simulink model "constFeed"  (R2022a)
settings: Solver=VariableStepAuto  StartTime=0.0  StopTime=240  RelTol=1e-3
settings Model: Creator=tomok  LastModifiedBy=tomok

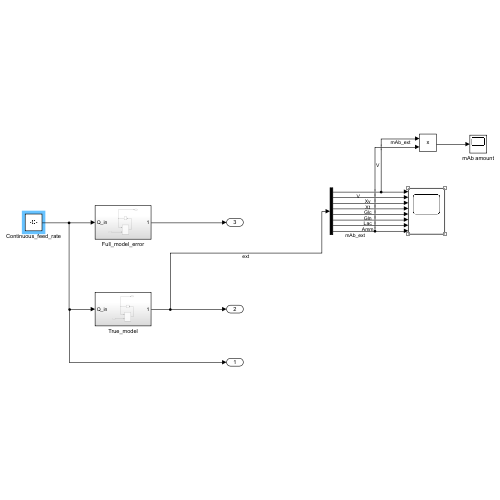
[thumbnail: Simulink's stored preview of the top-level diagram]
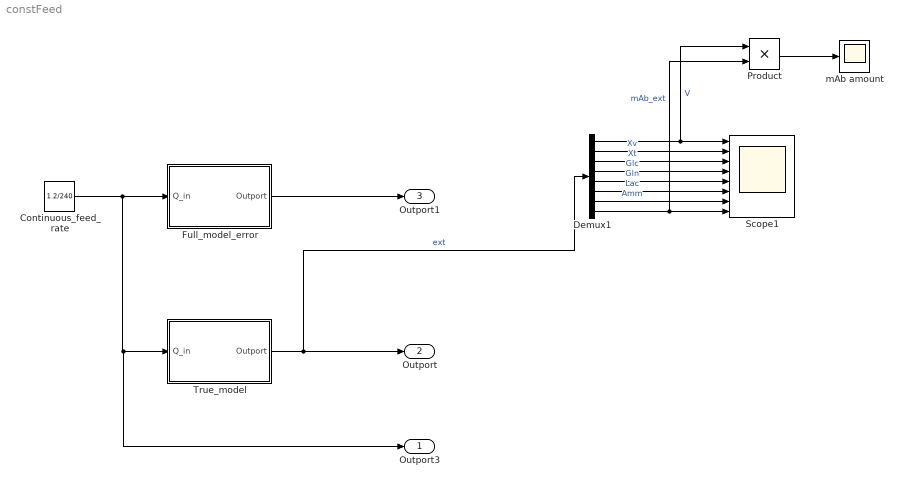
== system constFeed ==
  Continuous_feed_rate : Constant  Value=1.2/240
  Demux1 : Demux  Outputs=8
  Full_model_error : Subsystem
  Product : Product
  Scope1 : Scope  NumInputPorts=8
  True_model : Subsystem
  mAb amount : Scope
  Outport3 : Outport
  Outport : Outport  Port=2
  Outport1 : Outport  Port=3
  wires:
  Demux1/3 -> Scope1/3  "Xt"
  Demux1/6 -> Scope1/6  "Lac"
  Demux1/1 -> Product/1, Scope1/1  "V"
  Demux1/5 -> Scope1/5  "Gln"
  True_model/1(Outport) -> Demux1/1, Outport/1  "ext"
  Demux1/2 -> Scope1/2  "Xv"
  Demux1/4 -> Scope1/4  "Glc"
  Demux1/8 -> Product/2, Scope1/8  "mAb_ext"
  Demux1/7 -> Scope1/7  "Amm"
  Product/1 -> mAb amount/1
  Continuous_feed_rate/1 -> Outport3/1, True_model/1(Q_in), Full_model_error/1(Q_in)
  Full_model_error/1(Outport) -> Outport1/1

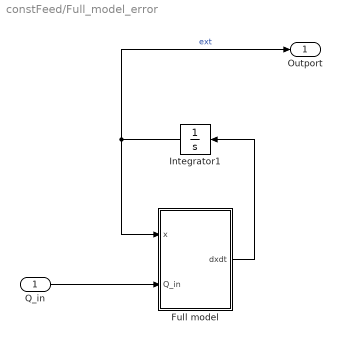
== system constFeed/Full_model_error ==
  Q_in : Inport
  Full model : MATLAB Function  TreatAsAtomicUnit=on
  Integrator1 : Integrator  InitialCondition=[0.8;2E+8;2E+8;25;4;0;0;0]  LimitOutput=on  LowerSaturationLimit=0
  Outport : Outport
  wires:
  Integrator1/1 -> Outport/1, Full model/1(x)  "ext"
  Full model/1(dxdt) -> Integrator1/1
  Q_in/1 -> Full model/2(Q_in)

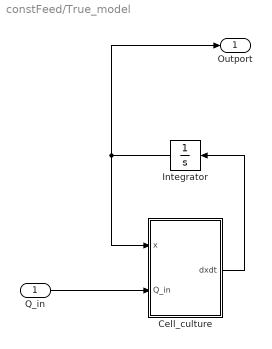
== system constFeed/True_model ==
  Q_in : Inport
  Cell_culture : MATLAB Function  TreatAsAtomicUnit=on
  Integrator : Integrator  InitialCondition=[0.8;2E+8;2E+8;25;4;0;0;0]  LimitOutput=on  LowerSaturationLimit=0
  Outport : Outport
  wires:
  Integrator/1 -> Outport/1, Cell_culture/1(x)
  Cell_culture/1(dxdt) -> Integrator/1
  Q_in/1 -> Cell_culture/2(Q_in)

== matlab function constFeed/Full_model_error/Full model ==
  data: dxdt output; x input; Q_in input
function dxdt = fcn(x,Q_in)
dxdt = deTremblay1992StateFcnError(x,Q_in);
end

== matlab function constFeed/True_model/Cell_culture ==
  data: dxdt output; x input; Q_in input
function dxdt = fcn(x,Q_in)
dxdt = deTremblay1992StateFcn(x,Q_in);
end
